simulink model "setup_ipm_resamplingtx"  (R2024b)
settings: Solver=FixedStepAuto  StartTime=0.0  StopTime=Runtime  FixedStep=1  RelTol=1e-3
undefined symbols (not defined in the file or in its folder): c_waveform_cfg
libraries: simulink x6
settings Model: Creator=jose.sanchez  LastModifiedBy=jose.sanchez
settings OptimizationCC: BlockReduction=off  ConditionallyExecuteInputs=off

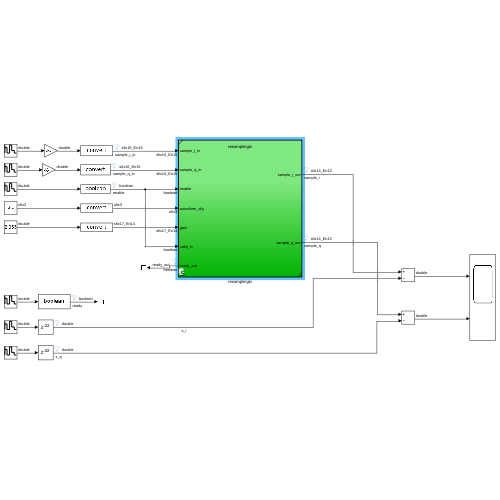
[thumbnail: Simulink's stored preview of the top-level diagram]
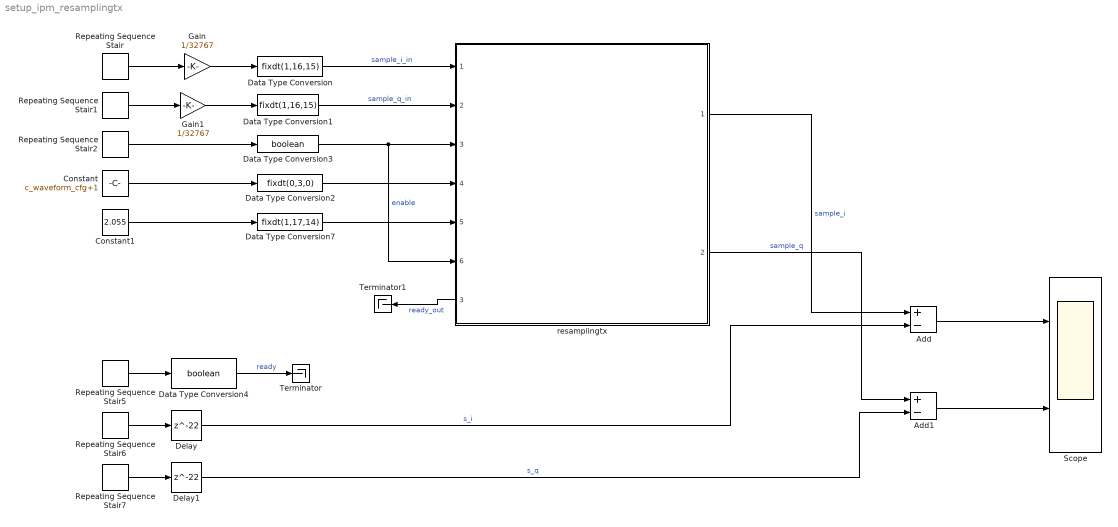
== system setup_ipm_resamplingtx ==
  Add : Sum  Inputs=+-
  Add1 : Sum  Inputs=+-
  Constant : Constant  Value=c_waveform_cfg+1  OutDataTypeStr=fixdt(0,2,0)
  Constant1 : Constant  Value=2.055
  Data Type Conversion : DataTypeConversion  OutDataTypeStr=fixdt(1,16,15)  SaturateOnIntegerOverflow=off  RndMeth=Floor
  Data Type Conversion1 : DataTypeConversion  OutDataTypeStr=fixdt(1,16,15)  SaturateOnIntegerOverflow=off  RndMeth=Floor
  Data Type Conversion2 : DataTypeConversion  OutDataTypeStr=fixdt(0,3,0)  SaturateOnIntegerOverflow=off  RndMeth=Floor
  Data Type Conversion3 : DataTypeConversion  OutDataTypeStr=boolean  SaturateOnIntegerOverflow=off  RndMeth=Floor
  Data Type Conversion4 : DataTypeConversion  OutDataTypeStr=boolean  SaturateOnIntegerOverflow=off  RndMeth=Floor
  Data Type Conversion7 : DataTypeConversion  OutDataTypeStr=fixdt(1,17,14)  SaturateOnIntegerOverflow=off  RndMeth=Floor
  Delay : Delay  DelayLength=22
  Delay1 : Delay  DelayLength=22
  Gain : Gain  Gain=1/32767
  Gain1 : Gain  Gain=1/32767
  Repeating Sequence Stair : simulink/Sources/Repeating Sequence Stair  OutValues=VHDL.din_i  tsamp=1  OutMin=[]  OutMax=[]  OutDataTypeStr=double  OutputDataTypeScalingMode=double  OutDataType=fixdt(0,8)  ConRadixGroup=Best Precision: Vector-wise  OutScaling=2^-12
  Repeating Sequence Stair1 : simulink/Sources/Repeating Sequence Stair  OutValues=VHDL.din_q  tsamp=1  OutMin=[]  OutMax=[]  OutDataTypeStr=double  OutputDataTypeScalingMode=double  OutDataType=fixdt(0,8)  ConRadixGroup=Best Precision: Vector-wise  OutScaling=2^-12
  Repeating Sequence Stair2 : simulink/Sources/Repeating Sequence Stair  OutValues=VHDL.valid  tsamp=1  OutMin=[]  OutMax=[]  OutDataTypeStr=double  OutputDataTypeScalingMode=double  OutDataType=fixdt(0,8)  ConRadixGroup=Best Precision: Vector-wise  OutScaling=2^-12
  Repeating Sequence Stair5 : simulink/Sources/Repeating Sequence Stair  OutValues=VHDL.ready  tsamp=1  OutMin=[]  OutMax=[]  OutDataTypeStr=double  OutputDataTypeScalingMode=double  OutDataType=fixdt(0,8)  ConRadixGroup=Best Precision: Vector-wise  OutScaling=2^-12
  Repeating Sequence Stair6 : simulink/Sources/Repeating Sequence Stair  OutValues=resampling.sample_i  tsamp=1  OutMin=[]  OutMax=[]  OutDataTypeStr=double  OutputDataTypeScalingMode=double  OutDataType=fixdt(0,8)  ConRadixGroup=Best Precision: Vector-wise  OutScaling=2^-12
  Repeating Sequence Stair7 : simulink/Sources/Repeating Sequence Stair  OutValues=resampling.sample_q  tsamp=1  OutMin=[]  OutMax=[]  OutDataTypeStr=double  OutputDataTypeScalingMode=double  OutDataType=fixdt(0,8)  ConRadixGroup=Best Precision: Vector-wise  OutScaling=2^-12
  Scope : Scope  NumInputPorts=2
  Terminator : Terminator
  Terminator1 : Terminator
  resamplingtx : Subsystem  ReferencedSubsystem=resamplingtx
      settings: PortSchema="{\"entries\":[{\"content\":{\"sides\":[{\"content\":{\"connectorIds\":[\"In1\",\"In2\",\"In3\",\"In4\",\"In5\",\"In6\",\"Out3\"]},\"type\":\"ConnectorPlacement.EquallySpacedRectSide\",\"uuid\":\"cf042d33-cf7c-44b7-94b5-89dedec5babb\"},{\"content\":{\"connectorIds\":[\"Out1\",\"Out2\"],\"side\":\"RIGHT\"},\"type\":\"ConnectorPlacement.EquallySpacedRectSide\",\"uuid\":\"78078c43-b521-49dc-8199-693957c84f97\"},{\"content\":{\"side\":\"TOP\"},\"type\":\"ConnectorPlacement.EquallySpacedRectSide\",\"uuid\":\"cf25d545-dc7a-4591-9aab-561bbc8f965a\"}]},\"type\":\"ConnectorPlacement.EquallySpacedConnector\",\"uuid\":\"b9ce6b16-b862-4bbf-b950-d3106e20ca77\"}],\"packageUris\":[\"http://schema.mathworks.com/mf0/Connector/R2020b\"],\"version\":\"1.0\"}"
  wires:
  Constant/1 -> Data Type Conversion2/1
  Data Type Conversion2/1 -> resamplingtx/4
  Gain1/1 -> Data Type Conversion1/1
  Repeating Sequence Stair2/1 -> Data Type Conversion3/1
  Repeating Sequence Stair/1 -> Gain/1
  Repeating Sequence Stair1/1 -> Gain1/1
  Gain/1 -> Data Type Conversion/1
  Data Type Conversion/1 -> resamplingtx/1  "sample_i_in"
  Data Type Conversion1/1 -> resamplingtx/2  "sample_q_in"
  Data Type Conversion3/1 -> resamplingtx/6, resamplingtx/3  "enable"
  Repeating Sequence Stair5/1 -> Data Type Conversion4/1
  Data Type Conversion4/1 -> Terminator/1  "ready"
  resamplingtx/3 -> Terminator1/1  "ready_out"
  resamplingtx/1 -> Add/1  "sample_i"
  Add/1 -> Scope/1
  Add1/1 -> Scope/2
  resamplingtx/2 -> Add1/1  "sample_q"
  Constant1/1 -> Data Type Conversion7/1
  Data Type Conversion7/1 -> resamplingtx/5
  Repeating Sequence Stair6/1 -> Delay/1
  Delay/1 -> Add/2  "s_i"
  Repeating Sequence Stair7/1 -> Delay1/1
  Delay1/1 -> Add1/2  "s_q"
